simulink model "OHC_NL_Boltzman_Function_fil"  (R2019b)
settings: Solver=VariableStepAuto  StartTime=0.0  StopTime=testtime  RelTol=1e-3
InitFcn:
  | OHC_NL_Boltzman_Test_Parameters
StopFcn:
  | Verify_OHC_NL_Boltzman_Function_fil
values from neighbouring files (symbols this model uses):
  Fs = 48e3    (= 48000)    [OHC_NL_Boltzman_Test_Parameters.m]
  s0 = 12.0    (= 12)    [OHC_NL_Boltzman_Test_Parameters.m]
  s1 = 5.0    (= 5)    [OHC_NL_Boltzman_Test_Parameters.m]
  shift = 1.0/(1.0+ohcasym)    (= 0.125)    [OHC_NL_Boltzman_Test_Parameters.m]
  x0 = s0*log((1.0/shift-1)/(1+exp(x1/s1)))    [OHC_NL_Boltzman_Test_Parameters.m]
  x1 = 5.0    (= 5)    [OHC_NL_Boltzman_Test_Parameters.m]
libraries: dspsrcs4 x2, simulink x1, fillib x1
settings Model: Creator=mblun  LastModifiedBy=t96f346
settings OptimizationCC: BlockReduction=off  ConditionallyExecuteInputs=off  DefaultParameterBehavior=Inlined
settings DebuggingCC: AlgebraicLoopMsg=error  InheritedTsInSrcMsg=none
settings HardwareCC: ProdBitPerPointer=32  ProdBitPerSizeT=32  ProdBitPerPtrDiffT=32  ProdLargestAtomicFloat=None  ProdIntDivRoundTo=Undefined  ProdEndianess=Unspecified  ProdWordSize=32  ProdHWDeviceType=ASIC/FPGA->ASIC/FPGA  TargetBitPerPointer=64  TargetBitPerSizeT=64  TargetBitPerPtrDiffT=64  TargetLongLongMode=on  TargetIntDivRoundTo=Zero  TargetEndianess=LittleEndian  TargetWordSize=64  TargetHWDeviceType=Custom Processor->MATLAB Host Computer  ProdEqTarget=off
settings SFSimCC: CustomCodeUndefinedFunction=UseInterfaceOnly

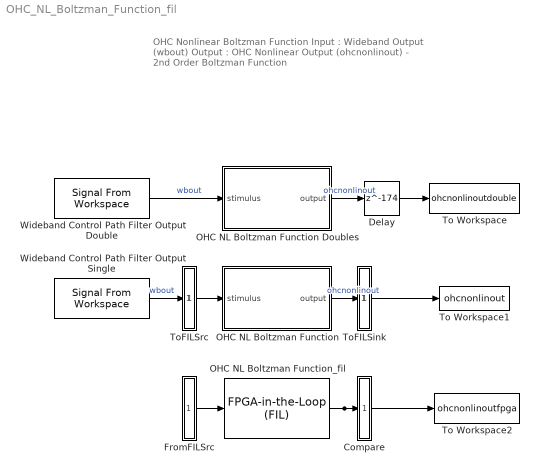
== system OHC_NL_Boltzman_Function_fil ==
  note: OHC Nonlinear Boltzman Function
      |
      | Input : Wideband Output (wbout)
      |
      | Output : OHC Nonlinear Output (ohcnonlinout)
      |
      | - 2nd Order Boltzman Function
  Compare : Subsystem
      mask Display: disp('')
  Delay : Delay  DelayLength=174
  FromFILSrc : Subsystem
      mask Display: disp('')
  OHC NL Boltzman Function : Subsystem
  OHC NL Boltzman Function Doubles : Subsystem
  OHC NL Boltzman Function_fil : fillib/FPGA-in-the-Loop (FIL)  ForceInterfaceUpdate=0.96489
      settings: SourceProductName=HDL Coder  SourceProductBaseCode=HD
  To Workspace : ToWorkspace  VariableName=ohcnonlinoutdouble  SampleTime=-1
      settings: Save2DSignal=2-D array (concatenate along first dimension)
  To Workspace1 : ToWorkspace  VariableName=ohcnonlinout  SampleTime=-1
      settings: Save2DSignal=2-D array (concatenate along first dimension)
  To Workspace2 : ToWorkspace  VariableName=ohcnonlinoutfpga  SampleTime=-1
      settings: Save2DSignal=2-D array (concatenate along first dimension)
  ToFILSink : Subsystem
      mask Display: disp('')
  ToFILSrc : Subsystem
      mask Display: disp('')
  Wideband Control Path Filter Output Double : dspsrcs4/Signal From Workspace  X=RxSignalDouble  Ts=1/Fs  nsamps=1  OutputAfterFinalValue=Setting to zero  ignoreOrWarnInputAndFrameLengths=off  OutputFrames=off
  Wideband Control Path Filter Output Single : dspsrcs4/Signal From Workspace  X=RxSignal  Ts=1/Fs  nsamps=1  OutputAfterFinalValue=Setting to zero  ignoreOrWarnInputAndFrameLengths=off  OutputFrames=off
  wires:
  Wideband Control Path Filter Output Double/1 -> OHC NL Boltzman Function Doubles/1(stimulus)  "wbout"
  OHC NL Boltzman Function Doubles/1(output) -> Delay/1  "ohcnonlinout"
  ToFILSrc/1(out1) -> OHC NL Boltzman Function/1(stimulus)
  OHC NL Boltzman Function/1(output) -> ToFILSink/1(in1)  "ohcnonlinout"
  Wideband Control Path Filter Output Single/1 -> ToFILSrc/1(in1)  "wbout"
  ToFILSink/1(out1) -> To Workspace1/1
  FromFILSrc/1(out1) -> OHC NL Boltzman Function_fil/1
  OHC NL Boltzman Function_fil/1 -> To Workspace2/1, Compare/1(in1)
  Delay/1 -> To Workspace/1

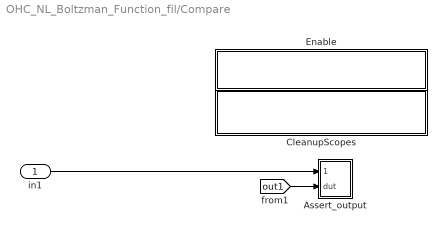
== system OHC_NL_Boltzman_Function_fil/Compare ==
  in1 : Inport
  Assert_output : Subsystem  mask{ToleranceValue=1e-07}
  CleanupScopes : Subsystem
      settings: OpenFcn=|
      | blkName = gcb; %self block
      | idx = regexp(blkName, '/CleanupScopes$', 'once');
      | blkParent = blkName(1:idx-1);
      | blks=find_system(blkParent, 'LookUnderMasks', 'all','blocktype', 'Scope');
      | for itr = 1:length(blks)
      | 	 hScopeCfg = get_param(blks{itr},'ScopeConfiguration');
      | 	 hScopeCfg.Visible = ~ hScopeCfg.Visible;
      | end
      | drawnow;
      mask Display: fprintf(message('hdlcoder:cosim:vnl_dblclick').getString());
  Enable : Subsystem
      settings: OpenFcn=|
      | blkName = gcb;
      | idx = regexp(blkName, '/Enable$', 'once');
      | blkParent = blkName(1:idx-1);
      | blks=find_system(blkParent, 'LookUnderMasks', 'all','blocktype', 'Assertion');
      | e = get_param(blks{1}, 'Enabled');
      | if strcmp(e, 'on'), f= 'off';, else, f = 'on';, end
      | for ii=1:length(blks), set_param(blks{ii}, 'Enabled', f);, end
      | set_param(gcb, 'MaskDisplay',['fprintf(message(''hdlcoder:cosim:vnl_dblclick_assertions'',','''',upper(e),'''',').getString())']);
      mask Display: fprintf(message('hdlcoder:cosim:vnl_dblclick_assertions','OFF').getString());
  wires:
  in1/1 -> Assert_output/1(cosim)
  [out1] -> Assert_output/2(dut)

== system OHC_NL_Boltzman_Function_fil/FromFILSrc ==
  dtc1 : DataTypeConversion  OutDataTypeStr=single  SaturateOnIntegerOverflow=on  RndMeth=Zero
  out1 : Outport
  wires:
  [in1] -> dtc1/1
  dtc1/1 -> out1/1

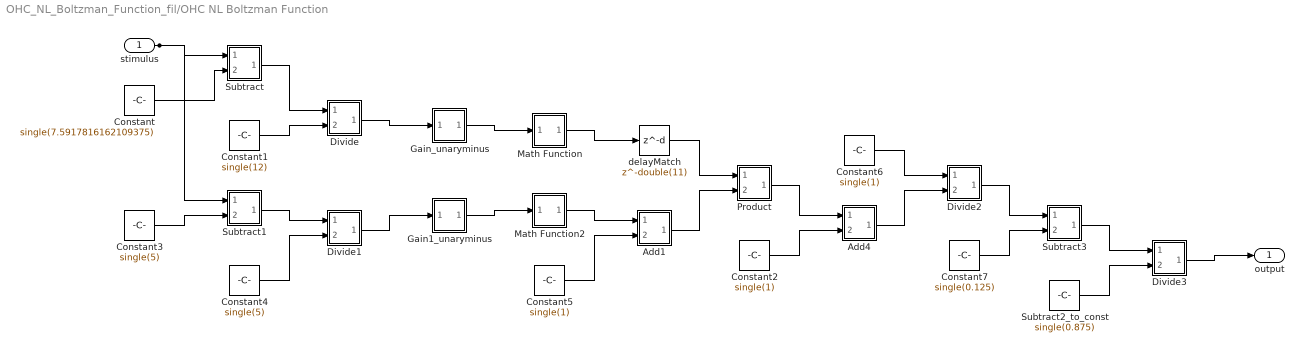
== system OHC_NL_Boltzman_Function_fil/OHC NL Boltzman Function ==
  stimulus : Inport  OutDataTypeStr=single  PortDimensions=1  SampleTime=2.08333333333333e-05
  Add1 : Subsystem
      mask Display: disp('NFP\nadd');
  Add4 : Subsystem
      mask Display: disp('NFP\nadd');
  Constant : Constant  Value=single(7.5917816162109375)  OutDataTypeStr=single  SampleTime=-1
  Constant1 : Constant  Value=single(12)  OutDataTypeStr=single  SampleTime=-1
  Constant2 : Constant  Value=single(1)  OutDataTypeStr=single  SampleTime=-1
  Constant3 : Constant  Value=single(5)  OutDataTypeStr=single  SampleTime=-1
  Constant4 : Constant  Value=single(5)  OutDataTypeStr=single  SampleTime=-1
  Constant5 : Constant  Value=single(1)  OutDataTypeStr=single  SampleTime=-1
  Constant6 : Constant  Value=single(1)  OutDataTypeStr=single  SampleTime=-1
  Constant7 : Constant  Value=single(0.125)  OutDataTypeStr=single  SampleTime=-1
  Divide : Subsystem
      mask Display: disp('NFP\nmul');
  Divide1 : Subsystem
      mask Display: disp('NFP\nmul');
  Divide2 : Subsystem
      mask Display: disp('NFP\nmul');
  Divide3 : Subsystem
      mask Display: disp('NFP\nmul');
  Gain1_unaryminus : Subsystem
      mask Display: disp('NFP\numinus');
  Gain_unaryminus : Subsystem
      mask Display: disp('NFP\numinus');
  Math Function : Subsystem
      mask Display: disp('NFP\nmath');
  Math Function2 : Subsystem
      mask Display: disp('NFP\nmath');
  Product : Subsystem
      mask Display: disp('NFP\nmul');
  Subtract : Subsystem
      mask Display: disp('NFP\nadd');
  Subtract1 : Subsystem
      mask Display: disp('NFP\nadd');
  Subtract2_to_const : Constant  Value=single(0.875)  OutDataTypeStr=single  SampleTime=-1
  Subtract3 : Subsystem
      mask Display: disp('NFP\nadd');
  delayMatch : Delay  DelayLength=double(11)  InitialCondition=0  SampleTime=2.08333333333333e-05
  output : Outport  VectorParamsAs1DForOutWhenUnconnected=off
  wires:
  Subtract3/1(Out1) -> Divide3/1(In1)
  Subtract1/1(Out1) -> Divide1/1(In1)
  Subtract/1(Out1) -> Divide/1(In1)
  Product/1(Out1) -> Add4/1(In1)
  Math Function2/1(Out1) -> Add1/1(In1)
  Math Function/1(Out1) -> delayMatch/1
  Divide3/1(Out1) -> output/1
  Divide2/1(Out1) -> Subtract3/1(In1)
  Divide1/1(Out1) -> Gain1_unaryminus/1(In1)
  Divide/1(Out1) -> Gain_unaryminus/1(In1)
  Add4/1(Out1) -> Divide2/2(In2)
  Add1/1(Out1) -> Product/2(In2)
  Gain1_unaryminus/1(Out1) -> Math Function2/1(In1)
  Gain_unaryminus/1(Out1) -> Math Function/1(In1)
  Subtract2_to_const/1 -> Divide3/2(In2)
  delayMatch/1 -> Product/1(In1)
  Constant7/1 -> Subtract3/2(In2)
  Constant6/1 -> Divide2/1(In1)
  Constant5/1 -> Add1/2(In2)
  Constant4/1 -> Divide1/2(In2)
  Constant3/1 -> Subtract1/2(In2)
  Constant2/1 -> Add4/2(In2)
  Constant1/1 -> Divide/2(In2)
  Constant/1 -> Subtract/2(In2)
  stimulus/1 -> Subtract/1(In1), Subtract1/1(In1)

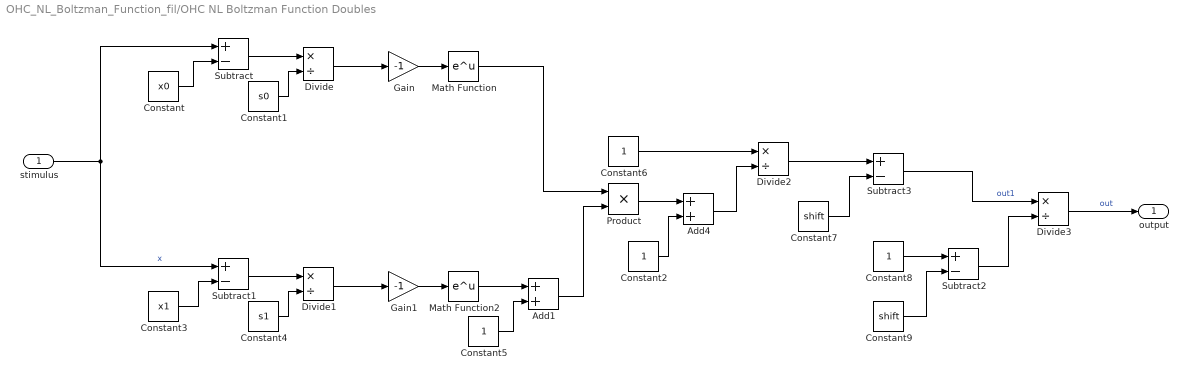
== system OHC_NL_Boltzman_Function_fil/OHC NL Boltzman Function Doubles ==
  stimulus : Inport
  Add1 : Sum
  Add4 : Sum
  Constant : Constant  Value=x0  SampleTime=-1
  Constant1 : Constant  Value=s0  SampleTime=-1
  Constant{2,5..6,8} (4 alike) : Constant  SampleTime=-1
  Constant3 : Constant  Value=x1  SampleTime=-1
  Constant4 : Constant  Value=s1  SampleTime=-1
  Constant7 : Constant  Value=shift  SampleTime=-1
  Constant9 : Constant  Value=shift  SampleTime=-1
  Divide{,1..3} (4 alike) : Product  Inputs=*/  SaturateOnIntegerOverflow=on  RndMeth=Zero
  Gain : Gain  Gain=-1
  Gain1 : Gain  Gain=-1
  Math Function : Math  SaturateOnIntegerOverflow=on
  Math Function2 : Math  SaturateOnIntegerOverflow=on
  Product : Product
  Subtract{,1..3} (4 alike) : Sum  Inputs=+-
  output : Outport  VectorParamsAs1DForOutWhenUnconnected=off
  wires:
  Constant/1 -> Subtract/2
  stimulus/1 -> Subtract1/1, Subtract/1  "x"
  Subtract/1 -> Divide/1
  Constant1/1 -> Divide/2
  Divide/1 -> Gain/1
  Gain/1 -> Math Function/1
  Constant3/1 -> Subtract1/2
  Subtract1/1 -> Divide1/1
  Constant4/1 -> Divide1/2
  Divide1/1 -> Gain1/1
  Gain1/1 -> Math Function2/1
  Math Function2/1 -> Add1/1
  Constant5/1 -> Add1/2
  Add1/1 -> Product/2
  Constant6/1 -> Divide2/1
  Divide2/1 -> Subtract3/1
  Constant7/1 -> Subtract3/2
  Subtract3/1 -> Divide3/1  "out1"
  Constant8/1 -> Subtract2/1
  Constant9/1 -> Subtract2/2
  Subtract2/1 -> Divide3/2
  Divide3/1 -> output/1  "out"
  Math Function/1 -> Product/1
  Product/1 -> Add4/1
  Constant2/1 -> Add4/2
  Add4/1 -> Divide2/2

== system OHC_NL_Boltzman_Function_fil/ToFILSink ==
  in1 : Inport
  out1 : Outport
  tag scope: out1=global
  wires:
  in1/1 -> out1/1, [out1]

== system OHC_NL_Boltzman_Function_fil/ToFILSrc ==
  in1 : Inport
  out1 : Outport
  tag scope: in1=global
  wires:
  in1/1 -> out1/1, [in1]

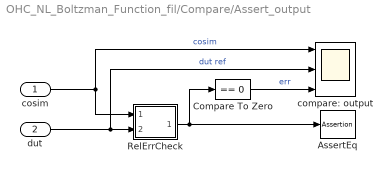
== system OHC_NL_Boltzman_Function_fil/Compare/Assert_output ==
  cosim : Inport
  dut : Inport  Port=2
  AssertEq : Assertion  StopWhenAssertionFail=off
  Compare To Zero : simulink/Logic and Bit Operations/Compare To Zero  relop===  OutDataTypeStr=boolean
  RelErrCheck : Subsystem
  compare: output : Scope  NumInputPorts=3
  wires:
  dut/1 -> compare: output/2, RelErrCheck/2(In2)  "dut ref"
  cosim/1 -> compare: output/1, RelErrCheck/1(In1)  "cosim"
  RelErrCheck/1(Out1) -> AssertEq/1, Compare To Zero/1
  Compare To Zero/1 -> compare: output/3  "err"

== system OHC_NL_Boltzman_Function_fil/Compare/CleanupScopes ==

== system OHC_NL_Boltzman_Function_fil/Compare/Enable ==

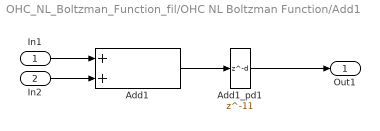
== system OHC_NL_Boltzman_Function_fil/OHC NL Boltzman Function/Add1 ==
  In1 : Inport
  In2 : Inport  Port=2
  Add1 : Sum  OutDataTypeStr=single  SampleTime=2.08333333333333e-05  SaturateOnIntegerOverflow=on  InputSameDT=on
  Add1_pd1 : Delay  DelayLength=11
  Out1 : Outport
  wires:
  Add1_pd1/1 -> Out1/1
  Add1/1 -> Add1_pd1/1
  In2/1 -> Add1/2
  In1/1 -> Add1/1

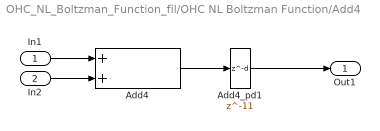
== system OHC_NL_Boltzman_Function_fil/OHC NL Boltzman Function/Add4 ==
  In1 : Inport
  In2 : Inport  Port=2
  Add4 : Sum  OutDataTypeStr=single  SampleTime=2.08333333333333e-05  SaturateOnIntegerOverflow=on  InputSameDT=on
  Add4_pd1 : Delay  DelayLength=11
  Out1 : Outport
  wires:
  Add4_pd1/1 -> Out1/1
  Add4/1 -> Add4_pd1/1
  In2/1 -> Add4/2
  In1/1 -> Add4/1

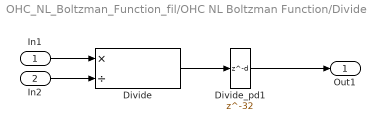
== system OHC_NL_Boltzman_Function_fil/OHC NL Boltzman Function/Divide ==
  In1 : Inport
  In2 : Inport  Port=2
  Divide : Product  Inputs=*/  OutDataTypeStr=single  SampleTime=2.08333333333333e-05  SaturateOnIntegerOverflow=on  RndMeth=Zero
  Divide_pd1 : Delay  DelayLength=32
  Out1 : Outport
  wires:
  Divide_pd1/1 -> Out1/1
  Divide/1 -> Divide_pd1/1
  In2/1 -> Divide/2
  In1/1 -> Divide/1

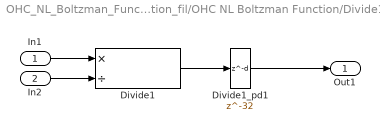
== system OHC_NL_Boltzman_Function_fil/OHC NL Boltzman Function/Divide1 ==
  In1 : Inport
  In2 : Inport  Port=2
  Divide1 : Product  Inputs=*/  OutDataTypeStr=single  SampleTime=2.08333333333333e-05  SaturateOnIntegerOverflow=on  RndMeth=Zero
  Divide1_pd1 : Delay  DelayLength=32
  Out1 : Outport
  wires:
  Divide1_pd1/1 -> Out1/1
  Divide1/1 -> Divide1_pd1/1
  In2/1 -> Divide1/2
  In1/1 -> Divide1/1

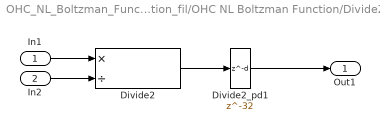
== system OHC_NL_Boltzman_Function_fil/OHC NL Boltzman Function/Divide2 ==
  In1 : Inport
  In2 : Inport  Port=2
  Divide2 : Product  Inputs=*/  OutDataTypeStr=single  SampleTime=2.08333333333333e-05  SaturateOnIntegerOverflow=on  RndMeth=Zero
  Divide2_pd1 : Delay  DelayLength=32
  Out1 : Outport
  wires:
  Divide2_pd1/1 -> Out1/1
  Divide2/1 -> Divide2_pd1/1
  In2/1 -> Divide2/2
  In1/1 -> Divide2/1

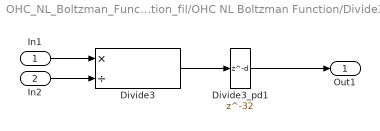
== system OHC_NL_Boltzman_Function_fil/OHC NL Boltzman Function/Divide3 ==
  In1 : Inport
  In2 : Inport  Port=2
  Divide3 : Product  Inputs=*/  OutDataTypeStr=single  SampleTime=2.08333333333333e-05  SaturateOnIntegerOverflow=on  RndMeth=Zero
  Divide3_pd1 : Delay  DelayLength=32
  Out1 : Outport
  wires:
  Divide3_pd1/1 -> Out1/1
  Divide3/1 -> Divide3_pd1/1
  In2/1 -> Divide3/2
  In1/1 -> Divide3/1

== system OHC_NL_Boltzman_Function_fil/OHC NL Boltzman Function/Gain1_unaryminus ==
  In1 : Inport
  Gain1_unaryminus : UnaryMinus  SampleTime=2.08333333333333e-05
  Out1 : Outport
  wires:
  Gain1_unaryminus/1 -> Out1/1
  In1/1 -> Gain1_unaryminus/1

== system OHC_NL_Boltzman_Function_fil/OHC NL Boltzman Function/Gain_unaryminus ==
  In1 : Inport
  Gain_unaryminus : UnaryMinus  SampleTime=2.08333333333333e-05
  Out1 : Outport
  wires:
  Gain_unaryminus/1 -> Out1/1
  In1/1 -> Gain_unaryminus/1

== system OHC_NL_Boltzman_Function_fil/OHC NL Boltzman Function/Math Function ==
  In1 : Inport
  Math Function : Math  SampleTime=2.08333333333333e-05  SaturateOnIntegerOverflow=on
  Math Function_pd1 : Delay  DelayLength=26
  Out1 : Outport
  wires:
  Math Function_pd1/1 -> Out1/1
  Math Function/1 -> Math Function_pd1/1
  In1/1 -> Math Function/1

== system OHC_NL_Boltzman_Function_fil/OHC NL Boltzman Function/Math Function2 ==
  In1 : Inport
  Math Function2 : Math  SampleTime=2.08333333333333e-05  SaturateOnIntegerOverflow=on
  Math Function2_pd1 : Delay  DelayLength=26
  Out1 : Outport
  wires:
  Math Function2_pd1/1 -> Out1/1
  Math Function2/1 -> Math Function2_pd1/1
  In1/1 -> Math Function2/1

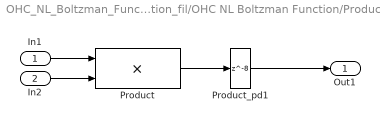
== system OHC_NL_Boltzman_Function_fil/OHC NL Boltzman Function/Product ==
  In1 : Inport
  In2 : Inport  Port=2
  Product : Product  Inputs=**  OutDataTypeStr=single  SampleTime=2.08333333333333e-05
  Product_pd1 : Delay  DelayLength=8
  Out1 : Outport
  wires:
  Product_pd1/1 -> Out1/1
  Product/1 -> Product_pd1/1
  In2/1 -> Product/2
  In1/1 -> Product/1

== system OHC_NL_Boltzman_Function_fil/OHC NL Boltzman Function/Subtract ==
  In1 : Inport
  In2 : Inport  Port=2
  Subtract : Sum  Inputs=+-  OutDataTypeStr=single  SampleTime=2.08333333333333e-05  SaturateOnIntegerOverflow=on  InputSameDT=on
  Subtract_pd1 : Delay  DelayLength=11
  Out1 : Outport
  wires:
  Subtract_pd1/1 -> Out1/1
  Subtract/1 -> Subtract_pd1/1
  In2/1 -> Subtract/2
  In1/1 -> Subtract/1

== system OHC_NL_Boltzman_Function_fil/OHC NL Boltzman Function/Subtract1 ==
  In1 : Inport
  In2 : Inport  Port=2
  Subtract1 : Sum  Inputs=+-  OutDataTypeStr=single  SampleTime=2.08333333333333e-05  SaturateOnIntegerOverflow=on  InputSameDT=on
  Subtract1_pd1 : Delay  DelayLength=11
  Out1 : Outport
  wires:
  Subtract1_pd1/1 -> Out1/1
  Subtract1/1 -> Subtract1_pd1/1
  In2/1 -> Subtract1/2
  In1/1 -> Subtract1/1

== system OHC_NL_Boltzman_Function_fil/OHC NL Boltzman Function/Subtract3 ==
  In1 : Inport
  In2 : Inport  Port=2
  Subtract3 : Sum  Inputs=+-  OutDataTypeStr=single  SampleTime=2.08333333333333e-05  SaturateOnIntegerOverflow=on  InputSameDT=on
  Subtract3_pd1 : Delay  DelayLength=11
  Out1 : Outport
  wires:
  Subtract3_pd1/1 -> Out1/1
  Subtract3/1 -> Subtract3_pd1/1
  In2/1 -> Subtract3/2
  In1/1 -> Subtract3/1

== system OHC_NL_Boltzman_Function_fil/Compare/Assert_output/RelErrCheck ==
  In1 : Inport
  In2 : Inport  Port=2
  "RelativeErrorCheck " : MATLAB Function  TreatAsAtomicUnit=on
  Out1 : Outport  VectorParamsAs1DForOutWhenUnconnected=off
  wires:
  In2/1 -> "RelativeErrorCheck "/2(R)
  In1/1 -> "RelativeErrorCheck "/1(P)
  "RelativeErrorCheck "/1(y) -> Out1/1

== matlab function OHC_NL_Boltzman_Function_fil/Compare/Assert_output/RelErrCheck/RelativeErrorCheck  ==
  data: P input; y output; R input; ToleranceValue parameter double
% Check if the relative error of R with respect to P is below
% ToleranceValue
% P, R are floating-point
function y = relErrCheck(P,R, ToleranceValue)
    tol = ToleranceValue;
    sz = numel(P);
    assert(sz == numel(R), 'Inputs P and R have different sizes.');
    y = false(1, sz);

    for ii=1:sz
        if (isnan(P(ii)) || isnan(R(ii)))
            if (isnan(P(ii)) && isnan(R(ii)))
                y(ii) = true;
            end
        elseif (isinf(P(ii)) || isinf(R(ii)))
            y(ii) = (P(ii) == R(ii));
        elseif (P(ii) == 0)
            y(ii) = (R(ii) == 0);
        else
            absdiff = abs(P(ii) - R(ii));
            relerr = absdiff/abs(P(ii));
            y(ii) = (relerr <= tol);
        end
    end
end
